simulink model "OPC_linea_transmision"  (R2018a)
settings: Solver=VariableStepAuto  StartTime=0.0  StopTime=inf  RelTol=1e-3
InitFcn:
  | SimulinkInit_linea_transmision
libraries: opclib x11, mpclib x1
settings Model: SimulationMode=accelerator  Creator=cmparedes  LastModifiedBy=AndrewB

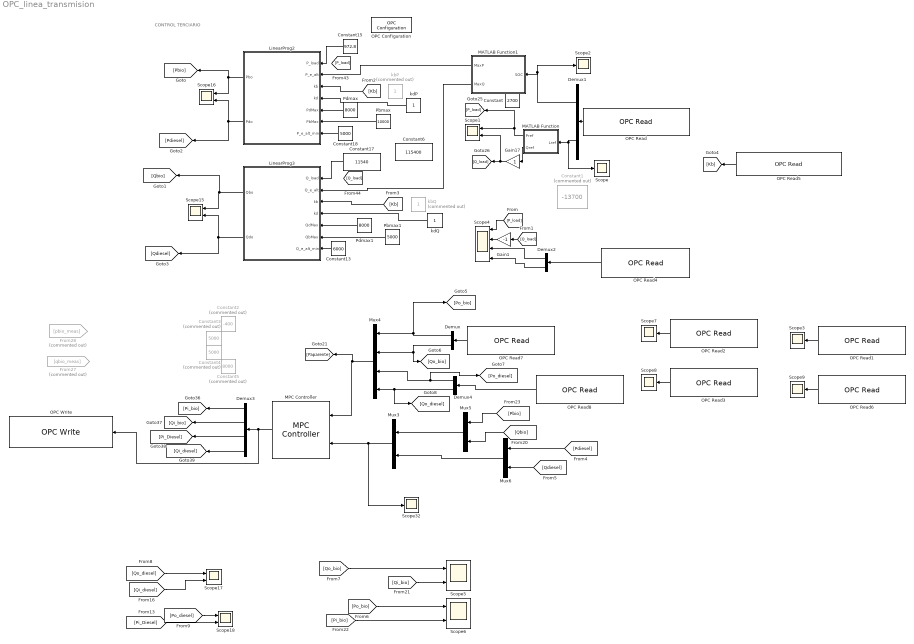
== system OPC_linea_transmision ==
  note: CONTROL TERCIARIO
  Constant : Constant  Value=2700
  Constant1 : Constant  Commented=on  Value=-13700
  Constant13 : Constant  Value=6000
  Constant15 : Constant  Value=972.8
  Constant17 : Constant  Value=11540
  Constant18 : Constant  Value=5000
  Constant2 : Constant  Commented=on  Value=-400
  Constant3 : Constant  Commented=on  Value=5000
  Constant4 : Constant  Commented=on  Value=5000
  Constant5 : Constant  Commented=on  Value=8000
  Constant6 : Constant  Value=115400
  Demux{,1..2,4} (4 alike) : Demux  Outputs=2
  Demux3 : Demux
  From27 : From  Commented=on  GotoTag=qbio_meas
  From28 : From  Commented=on  GotoTag=pbio_meas
  Gain1 : Gain  Gain=-1
  Gain17 : Gain
  LinearProg2 : MATLAB Function  TreatAsAtomicUnit=on  SystemSampleTime=1e-3
  LinearProg3 : MATLAB Function  TreatAsAtomicUnit=on  SystemSampleTime=1e-3
  MATLAB Function : MATLAB Function  TreatAsAtomicUnit=on
  MATLAB Function1 : MATLAB Function  TreatAsAtomicUnit=on
  MPC Controller : mpclib/MPC Controller  SCDEnableBlockLinearizationSpecification=on  mpcobj=mpcobj  is_multiple=0  enable_value=0  return_u0=off  updateMPCinCallerWorkspace=on  ref_from_ws=off  ref_signal_name=[]  ref_preview=off  md_from_ws=off  md_signal_name=[]  md_preview=off  from_project=off  project_file=MPCtask.mat  md_inport=off  mv_inport=off  cost_outport=off  return_sequence=off  return_qpstatus=off  return_state=off  state_inport=off  lims_inport=off  cc_inport=off  ywt_inport=off  is_designfromscratch=0  uwt_inport=off  duwt_inport=off  rhoeps_inport=off  uref_inport=off  n_ts=0.1  n_p=100  n_mv=4  n_md=0  n_ud=0  n_mo=4  n_uo=0  BlockDataType=double  SampleTimeInherited=off  switch_inport=off
  Mux3 : Mux  Inputs=2
  Mux4 : Mux
  Mux5 : Mux  Inputs=2
  Mux6 : Mux  Inputs=2
  OPC Configuration : opclib/OPC Configuration  opcServers=localhost/Kepware.KEPServerEX.V6/10  errMissingItems=Error  errReadWrite=Warn  errShutdown=Error  errRTViolation=Warn  rtEnable=on  speedup=1  showLatency=off  beingUsed=on
      settings: SourceProductName=OPC Toolbox  SourceProductBaseCode=OT
  OPC Read : opclib/OPC Read  serverHost=localhost  serverID=Kepware.KEPServerEX.V6  itemIDs=Carga_Reno_Channel.Carga.Group1.SOC, Carga_Reno_Channel.Carga.Group1.Lref  readMode=Synchronous (cache)  dataType=double  updateRate=0.1  showQual=off  showTS=off  tsMode=Seconds since start
      settings: SourceProductName=OPC Toolbox  SourceProductBaseCode=OT
  OPC Read1 : opclib/OPC Read  serverHost=localhost  serverID=Kepware.KEPServerEX.V6  itemIDs=Carga_Reno_Channel.Carga.Group1.Vload  readMode=Synchronous (cache)  dataType=double  updateRate=0.1  showQual=off  showTS=off  tsMode=Seconds since start
      settings: SourceProductName=OPC Toolbox  SourceProductBaseCode=OT
  OPC Read2 : opclib/OPC Read  serverHost=localhost  serverID=Kepware.KEPServerEX.V6  itemIDs=Bio_Channel.Bio.Group1.Ibio  readMode=Synchronous (cache)  dataType=double  updateRate=0.1  showQual=off  showTS=off  tsMode=Seconds since start
      settings: SourceProductName=OPC Toolbox  SourceProductBaseCode=OT
  OPC Read3 : opclib/OPC Read  serverHost=localhost  serverID=Kepware.KEPServerEX.V6  itemIDs=Diesel_Channel.Diesel.Group1.Idiesel  readMode=Synchronous (cache)  dataType=double  updateRate=0.1  showQual=off  showTS=off  tsMode=Seconds since start
      settings: SourceProductName=OPC Toolbox  SourceProductBaseCode=OT
  OPC Read4 : opclib/OPC Read  serverHost=localhost  serverID=Kepware.KEPServerEX.V6  itemIDs=Carga_Reno_Channel.Carga.Group1.Pm, Carga_Reno_Channel.Carga.Group1.Qm  readMode=Synchronous (cache)  dataType=double  updateRate=0.1  showQual=off  showTS=off  tsMode=Seconds since start
      settings: SourceProductName=OPC Toolbox  SourceProductBaseCode=OT
  OPC Read5 : opclib/OPC Read  serverHost=localhost  serverID=Kepware.KEPServerEX.V6  itemIDs=Carga_Reno_Channel.Carga.Group1.KB  readMode=Synchronous (cache)  dataType=double  updateRate=0.1  showQual=off  showTS=off  tsMode=Seconds since start
      settings: SourceProductName=OPC Toolbox  SourceProductBaseCode=OT
  OPC Read6 : opclib/OPC Read  serverHost=localhost  serverID=Kepware.KEPServerEX.V6  itemIDs=Carga_Reno_Channel.Carga.Group1.Ipv  readMode=Synchronous (cache)  dataType=double  updateRate=0.1  showQual=off  showTS=off  tsMode=Seconds since start
      settings: SourceProductName=OPC Toolbox  SourceProductBaseCode=OT
  OPC Read7 : opclib/OPC Read  serverHost=localhost  serverID=Kepware.KEPServerEX.V6  itemIDs=Bio_Channel.Bio.Group1.Pm, Bio_Channel.Bio.Group1.Qm  readMode=Synchronous (cache)  dataType=double  updateRate=0.1  showQual=off  showTS=off  tsMode=Seconds since start
      settings: SourceProductName=OPC Toolbox  SourceProductBaseCode=OT
  OPC Read8 : opclib/OPC Read  serverHost=localhost  serverID=Kepware.KEPServerEX.V6  itemIDs=Carga_Reno_Channel.Carga.Group1.Po_reno, Carga_Reno_Channel.Carga.Group1.Qo_reno  readMode=Synchronous (cache)  dataType=double  updateRate=0.1  showQual=off  showTS=off  tsMode=Seconds since start
      settings: SourceProductName=OPC Toolbox  SourceProductBaseCode=OT
  OPC Write : opclib/OPC Write  serverHost=localhost  serverID=Kepware.KEPServerEX.V6  itemIDs=Bio_Channel.Bio.Group1.Pref, Bio_Channel.Bio.Group1.Qref, Carga_Reno_Channel.Carga.Group1.Pi_reno, Carga_Reno_Channel.Carga.Group1.Qi_reno  writeMode=Synchronous  updateRate=0
      settings: SourceProductName=OPC Toolbox  SourceProductBaseCode=OT
  Pbmax : Constant  Value=10000
  Pbmax1 : Constant  Value=5000
  Pdmax : Constant  Value=8000
  Pdmax1 : Constant  Value=8000
  Scope{,2..3,7..9,32} (7 alike) : Scope
  Scope{1,5..6,15..18} (7 alike) : Scope  NumInputPorts=2
  Scope4 : Scope  NumInputPorts=4
  kbP : Constant  Commented=on
  kbQ : Constant  Commented=on
  kdP : Constant
  kdQ : Constant
  wires:
  LinearProg2/1(Pbo) -> [Pbio], Scope16/1
  LinearProg2/2(Pdo) -> [Pdiesel], Scope16/2
  Pdmax1/1 -> LinearProg3/5(QdMax)
  kdP/1 -> LinearProg2/4(kd)
  LinearProg3/2(Qdo) -> Scope15/2, [Qdiesel]
  MATLAB Function1/2(MaxQ) -> LinearProg3/2(Q_e_alt)
  LinearProg3/1(Qbo) -> [Qbio], Scope15/1
  MATLAB Function1/1(MaxP) -> LinearProg2/2(P_e_alt)
  kdQ/1 -> LinearProg3/4(kd)
  Gain17/1 -> Scope1/2, [Q_load]
  OPC Read/1 -> Demux1/1
  Demux1/1 -> Scope2/1, MATLAB Function1/1(SOC)
  MATLAB Function/2(Qref) -> Gain17/1
  MATLAB Function/1(Pref) -> Scope1/1, [P_load]
  OPC Read4/1 -> Demux2/1
  Demux2/1 -> Scope4/3
  Demux2/2 -> Scope4/4
  [P_load] -> Scope4/1
  Demux1/2 -> Scope/1, MATLAB Function/1(Lref)
  Gain1/1 -> Scope4/2
  [Q_load] -> Gain1/1
  OPC Read5/1 -> [Kb]
  [Kb] -> LinearProg3/3(kb)
  [Kb] -> LinearProg2/3(kb)
  Constant15/1 -> LinearProg2/1(P_load)
  Constant17/1 -> LinearProg3/1(Q_load)
  Pdmax/1 -> LinearProg2/5(PdMax)
  Pbmax/1 -> LinearProg2/6(PbMax)
  Constant18/1 -> LinearProg2/7(P_e_alt_min)
  Pbmax1/1 -> LinearProg3/6(QbMax)
  Constant13/1 -> LinearProg3/7(Q_e_alt_min)
  Mux3/1 -> Scope32/1, MPC Controller/2
  Demux/2 -> Mux4/2, [Qo_bio]
  Demux3/4 -> [Qi_diesel]
  MPC Controller/1 -> OPC Write/1, Demux3/1
  Demux3/3 -> [Pi_Diesel]
  Mux6/1 -> Mux3/2
  Demux4/2 -> [Qo_diesel], Mux4/4
  Demux3/1 -> [Pi_bio]
  Demux3/2 -> [Qi_bio]
  Mux4/1 -> [Paparente], MPC Controller/1
  Demux/1 -> Mux4/1, [Po_bio]
  Mux5/1 -> Mux3/1
  [Pbio] -> Mux5/1
  [Qbio] -> Mux5/2
  [Pdiesel] -> Mux6/1
  [Qdiesel] -> Mux6/2
  [Qo_diesel] -> Scope17/1
  [Qi_bio] -> Scope5/2
  [Po_diesel] -> Scope18/1
  [Pi_Diesel] -> Scope18/2
  [Qi_diesel] -> Scope17/2
  [Pi_bio] -> Scope6/2
  [Qo_bio] -> Scope5/1
  [Po_bio] -> Scope6/1
  OPC Read1/1 -> Scope3/1
  OPC Read2/1 -> Scope7/1
  OPC Read3/1 -> Scope8/1
  OPC Read6/1 -> Scope9/1
  OPC Read7/1 -> Demux/1
  OPC Read8/1 -> Demux4/1
  Demux4/1 -> [Po_diesel], Mux4/3

== matlab function OPC_linea_transmision/MATLAB Function ==
  data: Lref input; Pref output; Qref output
function [Pref,Qref] = fcn(Lref)

Pref = 1000;
Qref = 1000;%sqrt(Lref^2 - Pref^2);

== matlab function OPC_linea_transmision/LinearProg2 ==
  data: P_load input; Pbo output; P_e_alt input; kb input; kd input; PdMax input; PbMax input; Pdo output; P_e_alt_min input
function [Pbo, Pdo] = fcn(P_load, P_e_alt, kb, kd, PdMax, PbMax, P_e_alt_min)

% P_load es la potencia que se requiere en la carga.

% P_e_alt es la potencia estimada de generacion de las energias
% alternativas

% kb y kd son los pesos de las funcion de costo.

% las salidas son las potencias optimas para bio y diesel

Pb=0;
Pd=0;

D_P_e_alt = P_e_alt - P_e_alt_min; % superaavit de energia alternativa.

flagDelt = 0;

if(D_P_e_alt >= P_load)
    flagDelt = 1;
end
   

if(flagDelt==0)
    P_trad = P_load - D_P_e_alt;
    % flag: variable que indica si tiene sentido evaluar los
    % if's que se encuentran mas adelante. es decir, si flag = 0 
    % despues del primer if entonces NO se le esta pidiendo al sistema
    % mas potencia de la que puede generar y portanto el problema de 
    % optimizacion lineal tiene sentido.
    % entonces 
    flag=0;

    if(P_trad>PdMax+PbMax)
        Pd=PdMax;
        Pb=PbMax;
        flag=1;
    end

    % si ambas energias tienen el mismo factor de costo.
    if(kd==kb && flag==0)
        Pb=P_trad/2;
        Pd=P_trad/2;
    end

    % si la energia diesel es mas cara que la biomasa.
    if(kd>kb && flag==0)
        if(P_trad<=PbMax)
            Pb=P_trad;
            Pd=0;
        else
            Pb=PbMax;
            Pd=P_trad-PbMax;
        end
    end

    % si la biomasa es mas cara que la diesel.
    if(kd<kb && flag==0)
        if(P_trad<=PdMax)
            Pd=P_trad;
            Pb=0;
        else
            Pd=PdMax;
            Pb=P_trad-PdMax;
        end
    end
end

Pbo=Pb;
Pdo=Pd;

== matlab function OPC_linea_transmision/LinearProg3 ==
  data: Q_load input; Qbo output; Q_e_alt input; kb input; kd input; QdMax input; QbMax input; Qdo output; Q_e_alt_min input
function [Qbo, Qdo] = fcn(Q_load, Q_e_alt, kb, kd, QdMax, QbMax, Q_e_alt_min)

% Q_load es la Qotencia que se requiere en la carga.

% Q_e_alt es la Qotencia estimada de generacion de las energias
% alternativas

% kb y kd son los Qesos de las funcion de costo.

% las salidas son las Qotencias oQtimas Qara bio y diesel

Qb=0;
Qd=0;

D_Q_e_alt = Q_e_alt - Q_e_alt_min; % suQeraavit de energia alternativa.

flagDelt = 0;

if(D_Q_e_alt >= Q_load)
    flagDelt = 1;
end
   

if(flagDelt==0)
    Q_trad = Q_load - D_Q_e_alt;
    % flag: variable que indica si tiene sentido evaluar los
    % if's que se encuentran mas adelante. es decir, si flag = 0 
    % desQues del Qrimer if entonces NO se le esta Qidiendo al sistema
    % mas Qotencia de la que Quede generar y Qortanto el Qroblema de 
    % oQtimizacion lineal tiene sentido.
    % entonces 
    flag=0;

    if(Q_trad>QdMax+QbMax)
        Qd=QdMax;
        Qb=QbMax;
        flag=1;
    end

    % si ambas energias tienen el mismo factor de costo.
    if(kd==kb && flag==0)
        Qb=Q_trad/2;
        Qd=Q_trad/2;
    end

    % si la energia diesel es mas cara que la biomasa.
    if(kd>kb && flag==0)
        if(Q_trad<=QbMax)
            Qb=Q_trad;
            Qd=0;
        else
            Qb=QbMax;
            Qd=Q_trad-QbMax;
        end
    end

    % si la biomasa es mas cara que la diesel.
    if(kd<kb && flag==0)
        if(Q_trad<=QdMax)
            Qd=Q_trad;
            Qb=0;
        else
            Qd=QdMax;
            Qb=Q_trad-QdMax;
        end
    end
end

Qbo=Qb;
Qdo=Qd;

== matlab function OPC_linea_transmision/MATLAB Function1 ==
  data: SOC input; MaxP output; MaxQ output
function [MaxP, MaxQ] = fcn(SOC)


%  funcion que calcula la potencia maxima que puede suministrar las fuentes
%  renovables deacuerdo a la cantidad de carga que hay almancenada en la
%  bateria. esta va de 0 a 100%


% estoc valores que aparecen a continuacion se pusieron de manera
% arbitraria. corresponde a una persona con especialidad en la parte de
% potencia electrica determinar el verdadero algoritmo para hallar la
% potencia que deberia suministrar el nodo de energia renovable deacuerdo a
% la carga de la bateria.

MaxP = 0;
MaxQ = 0;

if( SOC >= 90 )
    MaxP = 500;
    MaxQ = 10000;
end

if( SOC <= 90 )
    MaxP = 200;
    MaxQ = 8000;
end

if( SOC <= 70 )
    MaxP = 70;
    MaxQ = 4000;
end

if( SOC <= 60 )
    MaxP = 50;
    MaxQ = 1000;
end
